simulink model "Diesel_NGCHP_v2"  (Simulink 8.1)
settings: Solver=ode4  StartTime=0.0  StopTime=inf  FixedStep=Ts  MaxStep=1e-3  RelTol=1e-3
model workspace (MAT data in the model file):
  op_snapshot1 : opcond.OperatingPoint (value not decoded)
PostLoadFcn:
  | Diesel_NGCHP_init;
InitFcn:
  | Diesel_NGCHP_init;
values from neighbouring files (symbols this model uses):
  Ts = 100E-6    (= 0.0001)    [Diesel_NGCHP_init.m]
undefined symbols (not defined in the file or in its folder): cable_spec, Diesel_Genset_lib, DiscIntNeverNeededParam, fdesignblkfcn, gcbh, Left, NG_CHP, NG_CHP_lib, ph, type, V
libraries: simulink x16, rtio_opalrt_common x15, powerlib x11, NG_Genset_lib x6, cables_lib x6, rtlab x5, simulink_extras x5, breaker_lib x4, rteventslib x4, powerlib_extras x3, discretizing x2, ssn_lib x2
(part 1 of 3)
settings Model: ARTEMISmethode_block_infos=$$__separator__$$Diesel_NGCHP_v2/ARTEMIS Guide$$__separator__$$  Creator=RE25624  LastModifiedBy=re25624  BufferReuse=off
settings SolverCC: ZeroCrossAlgorithm=Adaptive
settings DataIOCC: ExternalInput=getinputstruct(op_snapshot1)  InitialState=getstatestruct(op_snapshot1)  LimitDataPoints=off  MaxDataPoints=90060  SignalLoggingSaveFormat=Dataset  SaveOutput=off  SignalLogging=off  DSMLogging=off  SaveTime=off  OutputSaveName=result
settings OptimizationCC: BlockReduction=off  OptimizeBlockIOStorage=off  BufferReuse=off  ExpressionFolding=off  LocalBlockOutputs=off
settings DebuggingCC: MaxConsecutiveZCsMsg=warning  IgnoredZcDiagnostic=none  SolverPrmCheckMsg=none  MultiTaskRateTransMsg=warning  FcnCallInpInsideContextMsg=EnableAllAsWarning  FrameProcessingCompatibilityMsg=error  ModelReferenceExtraNoncontSigs=warning  StrictBusMsg=None
settings ModelReferenceCC: UpdateModelReferenceTargets=IfOutOfDate
settings SFSimCC: SFSimEcho=off
settings GRTTargetCC: CodeReplacementLibrary=C89/C90 (ANSI)

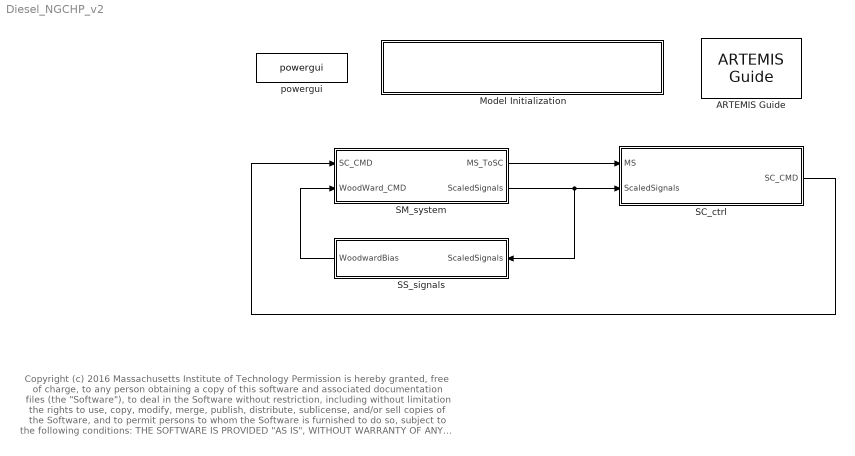
== system Diesel_NGCHP_v2 ==
  note: Copyright (c) 2016 Massachusetts Institute of Technology
      | Permission is hereby granted, free of charge, to any person obtaining a copy of this software and associated documentation files (the "Software"), to deal
      | in the Software without restriction, including without limitation the rights to use, copy, modify, merge, publish, distribute, sublicense, and/or sell copies of the
      | Software, and to permit persons to whom the Software is furnished to do so, subject to the following conditions:
      |
      | THE SOFTWARE IS PROVIDED "AS IS", WITHOUT WARRANTY OF ANY KIND, EXPRESS OR IMPLIED, INCLUDING BUT NOT LIMITED TO THE
      | WARRANTIES OF MERCHANTABILITY, FITNESS FOR A PARTICULAR PURPOSE AND NONINFRINGEMENT. IN NO EVENT SHALL THE AUTHORS
      | OR COPYRIGHT HOLDERS BE LIABLE FOR ANY CLAIM, DAMAGES OR OTHER LIABILITY, WHETHER IN AN ACTION OF CONTRACT, TORT OR
      | OTHERWISE, ARISING FROM, OUT OF OR IN CONNECTION WITH THE SOFTWARE OR THE USE OR OTHER DEALINGS IN THE SOFTWARE.
  ARTEMIS Guide : artemis/ARTEMIS/ARTEMIS Guide  Tag=FTSSmethode_opal_4hx0r99  Description=5.0_z1  lock=on  Ts=Ts  opt=art5  dyna=off  nb_perm=4  RT_fullcomp=off  ssn=on  ssn_itvc=off  ssn_ivic=off  ssn_ext=off  ssn_solver=Art5 with Backward Euler nodal interface  ssn_impulse=off  ssn_quasimpulse=off  ssn_impulse_loop=2  paraExtinctionThy=off  Thy_Impulse=on  dtc=Off  dtc_opt=normal  ao=on  simtype=off  ct_mac=off  lin_mov=off  lsp=[0.001 2]  spike_skip=Disabled  dtc_extra=1  dtc_sws=normal  dtc_pied=0.5  SPSRulesBlock=SPSRules  tre=on  ctmm=off  LF=off  dpl_type=ARTEMiS DPL  rlc_type=off  custom_type=off  para=on  ssn_ImpulseLoopBlockedStateUpdate=2  ssn_mov_iter_number=5  ssn_switch_iter_number=5
  Model Initialization : Subsystem  AncestorBlock=artemis/Tools /Misc/Model Initialization  mask(Model Functions){InitFcnX=Diesel_NGCHP_init;, prel=off, posl=on, inif=on, strf=off}
      mask prompts: InitFcnX "Initialisation"; prel "Preload Function"; posl "PostLoad Function"; inif "InitFcn"; strf "StartFcn"
      mask init:
      | currentBlock = gcb;
      | root = bdroot(currentBlock);
      | 
      | 
      | if ~strcmp(get_param(root,'BlockDiagramType'),'library')
      |     if prel==1
      |         set_param(root, 'PreLoadFcn', InitFcnX);
      |     else
      |         set_param(root, 'PreLoadFcn', '');
      |     end
      |     if inif==1
      |         set_param(root, 'InitFcn', InitFcnX);
      |     else
      |         set_param(root, 'InitFcn', '');
      |     end
      |     if strf==1
      |         set_param(root, 'StartFcn', InitFcnX);
      |     else
      |         set_param(root, 'StartFcn', '');
      |     end
      |     if posl==1
      |         set_param(root, 'PostLoadFcn', InitFcnX);
      |     else
      |         set_param(root, 'PostLoadFcn', '');
      |     end
      | end
      | 
      | pos = get_param(currentBlock, 'Position');
      | width = pos(3) - pos(1); height = pos(4) - pos(2);
      | txt = [ upper(root) '\n' '- InitFcn. . . . . '  get_param(root, 'InitFcn') ];
      settings: CopyFcn=set_param(gcb,'LinkStatus','inactive')
      mask Display: text(5, height*0.5, txt, 'horizontalAlignment', 'left', 'verticalAlignment', 'middle') ;
  SC_ctrl : Subsystem
  SM_system : Subsystem
  SS_signals : Subsystem
  powergui : powerlib/powergui  Priority=2  SimulationMode=Discrete  SolverType=Tustin  SampleTime=Ts  frequency=60  SPID=off  DisableSnubberDevices=off  DisableRonSwitches=off  DisableVfSwitches=off  SwTol=0  Interpol=off  DisplayEquations=off  frequencyindice=0  Pbase=100e6  ErrMax=1e-4  Iterations=50  UnitsV=kV  UnitsW=MW  FunctionMessages=off  echomessages=off  HookPort=off  EnableUseOfTLC=off  x0status=blocks  RestoreLinks=warning  ResistiveCurrentMeasurement=off  Frange=logspace(0,3,50)  Ylog=off  Xlog=off  ShowGrid=off  save=off  variable=ZData  structure=0  ZoomFFT=on  StartTime=0.0  cycles=2  DisplayStyle=off  fundamental=60  FreqAxis=off  MaxFrequency=1000  frequencyindicesteady=1  RmsSteady=1  display=off  Ts=0  methode=off
  wires:
  SM_system/1(MS_ToSC) -> SC_ctrl/1(MS)
  SC_ctrl/1(SC_CMD) -> SM_system/1(SC_CMD)
  SM_system/2(ScaledSignals) -> SS_signals/1(ScaledSignals), SC_ctrl/2(ScaledSignals)
  SS_signals/1(WoodwardBias) -> SM_system/2(WoodWard_CMD)

== system Diesel_NGCHP_v2/Model Initialization ==

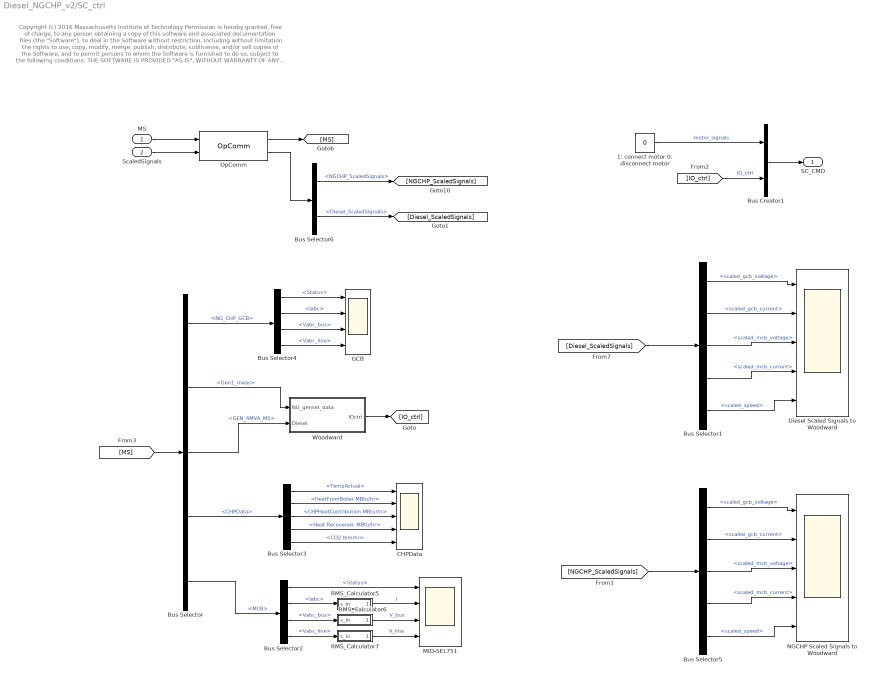
== system Diesel_NGCHP_v2/SC_ctrl ==
  note: Copyright (c) 2016 Massachusetts Institute of Technology
      | Permission is hereby granted, free of charge, to any person obtaining a copy of this software and associated documentation files (the "Software"), to deal
      | in the Software without restriction, including without limitation the rights to use, copy, modify, merge, publish, distribute, sublicense, and/or sell copies of the
      | Software, and to permit persons to whom the Software is furnished to do so, subject to the following conditions:
      |
      | THE SOFTWARE IS PROVIDED "AS IS", WITHOUT WARRANTY OF ANY KIND, EXPRESS OR IMPLIED, INCLUDING BUT NOT LIMITED TO THE
      | WARRANTIES OF MERCHANTABILITY, FITNESS FOR A PARTICULAR PURPOSE AND NONINFRINGEMENT. IN NO EVENT SHALL THE AUTHORS
      | OR COPYRIGHT HOLDERS BE LIABLE FOR ANY CLAIM, DAMAGES OR OTHER LIABILITY, WHETHER IN AN ACTION OF CONTRACT, TORT OR
      | OTHERWISE, ARISING FROM, OUT OF OR IN CONNECTION WITH THE SOFTWARE OR THE USE OR OTHER DEALINGS IN THE SOFTWARE
  MS : Inport
  ScaledSignals : Inport  Port=2
  1: connect motor 0: disconnect motor : Constant  Value=0
  Bus Creator1 : BusCreator  Inputs=2
  Bus Selector : BusSelector  OutputSignals=NG_CHP_MS.NG_CHP_GCB,NG_CHP_MS.Gen1_meas,GEN_4MVA_MS,NG_CHP_MS.CHPData,MCB
  Bus Selector1 : BusSelector  OutputSignals=scaled_gcb_voltage,scaled_gcb_current,scaled_mcb_voltage,scaled_mcb_current,scaled_speed
  Bus Selector2 : BusSelector  OutputSignals=Status,Iabc,Vabc_bus,Vabc_line
  Bus Selector3 : BusSelector  OutputSignals=TempActual,HeatFromBoiler MBtu/hr,CHPHeatContribution MBtu/hr,Thermal data.Heat Recovered; MBtu/hr,Thermal data.CO2 lbm/hr
  Bus Selector4 : BusSelector  OutputSignals=Status,Iabc,Vabc_bus,Vabc_line
  Bus Selector5 : BusSelector  OutputSignals=scaled_gcb_voltage,scaled_gcb_current,scaled_mcb_voltage,scaled_mcb_current,scaled_speed
  Bus Selector6 : BusSelector  OutputSignals=NGCHP_ScaledSignals,Diesel_ScaledSignals
  CHPData : Scope  NumInputPorts=5
      settings: ShowLegends=on  TimeRange=10  YMin=19.11~0~-1~1.37518~932.98  YMax=19.2~5.5~1~1.37533~933.08  SaveName=ScopeData5
  Diesel Scaled Signals to Woodward : Scope  NumInputPorts=5
      settings: YMin=-17.5~-0.000175~-17.5~-45~-5  YMax=17.5~0.000175~17.5~45~10  SaveName=ScopeData7
  GCB : Scope  NumInputPorts=4
      settings: ShowLegends=on  TimeRange=0.02  YMin=-1~-0.00015~-0.0025~-12500  YMax=1~0.00015~0.0025~12500
  MID-SEL751 : Scope  NumInputPorts=4
      settings: ShowLegends=on  TimeRange=1  YMin=0.95~-225~-12000~-12000  YMax=1.05~225~12000~12000  SaveName=ScopeData2
  NGCHP Scaled Signals to Woodward : Scope  NumInputPorts=5
      settings: YMin=-17.5~-0.000175~-17.5~-45~-5  YMax=17.5~0.000175~17.5~45~10  SaveName=ScopeData8
  OpComm : rtlab/OpComm  nbport=2  groupe_acq=1  subsys_rate=0  st=0  Synchronization=on  Interpolation=on  Threshold=1.0  Missed_Data=off  Sim_Time=off  Samples=off  dynSigOut=off  from_console=0  warning_done=off  writeOpCommFile=off  Offset=off
  RMS_Calculator5 : Subsystem
  RMS_Calculator6 : Subsystem
  RMS_Calculator7 : Subsystem
  Woodward : Subsystem
  SC_CMD : Outport
  wires:
  OpComm/1 -> [MS]
  MS/1 -> OpComm/1
  Woodward/1(IOctrl) -> [IO_ctrl]
  Bus Selector4/1 -> GCB/1  "<Status>"
  Bus Selector4/2 -> GCB/2  "<Iabc>"
  Bus Selector4/3 -> GCB/3  "<Vabc_bus>"
  Bus Selector4/4 -> GCB/4  "<Vabc_line>"
  Bus Selector/1 -> Bus Selector4/1  "<NG_CHP_GCB>"
  Bus Selector/2 -> Woodward/1(NG_genset_data)  "<Gen1_meas>"
  [MS] -> Bus Selector/1
  Bus Selector/4 -> Bus Selector3/1  "<CHPData>"
  Bus Selector3/1 -> CHPData/1  "<TempActual>"
  Bus Selector3/5 -> CHPData/5  "<CO2 lbm/hr>"
  Bus Selector3/2 -> CHPData/2  "<HeatFromBoiler MBtu/hr>"
  Bus Selector3/3 -> CHPData/3  "<CHPHeatContribution MBtu/hr>"
  Bus Selector3/4 -> CHPData/4  "<Heat Recovered; MBtu/hr>"
  Bus Creator1/1 -> SC_CMD/1
  1: connect motor 0: disconnect motor/1 -> Bus Creator1/1  "motor_signals"
  Bus Selector2/1 -> MID-SEL751/1  "<Status>"
  Bus Selector2/2 -> RMS_Calculator5/1(s_in)  "<Iabc>"
  Bus Selector2/3 -> RMS_Calculator6/1(s_in)  "<Vabc_bus>"
  Bus Selector2/4 -> RMS_Calculator7/1(s_in)  "<Vabc_line>"
  RMS_Calculator5/1(s_out) -> MID-SEL751/2  "I"
  RMS_Calculator6/1(s_out) -> MID-SEL751/3  "V_bus"
  RMS_Calculator7/1(s_out) -> MID-SEL751/4  "V_line"
  Bus Selector/5 -> Bus Selector2/1  "<MCB>"
  Bus Selector/3 -> Woodward/2(Diesel)  "<GEN_4MVA_MS>"
  [IO_ctrl] -> Bus Creator1/2  "IO_ctrl"
  Bus Selector1/1 -> Diesel Scaled Signals to Woodward/1  "<scaled_gcb_voltage>"
  Bus Selector1/2 -> Diesel Scaled Signals to Woodward/2  "<scaled_gcb_current>"
  Bus Selector1/3 -> Diesel Scaled Signals to Woodward/3  "<scaled_mcb_voltage>"
  Bus Selector1/4 -> Diesel Scaled Signals to Woodward/4  "<scaled_mcb_current>"
  Bus Selector1/5 -> Diesel Scaled Signals to Woodward/5  "<scaled_speed>"
  [Diesel_ScaledSignals] -> Bus Selector1/1
  Bus Selector5/1 -> NGCHP Scaled Signals to Woodward/1  "<scaled_gcb_voltage>"
  Bus Selector5/2 -> NGCHP Scaled Signals to Woodward/2  "<scaled_gcb_current>"
  Bus Selector5/3 -> NGCHP Scaled Signals to Woodward/3  "<scaled_mcb_voltage>"
  Bus Selector5/4 -> NGCHP Scaled Signals to Woodward/4  "<scaled_mcb_current>"
  Bus Selector5/5 -> NGCHP Scaled Signals to Woodward/5  "<scaled_speed>"
  [NGCHP_ScaledSignals] -> Bus Selector5/1
  OpComm/2 -> Bus Selector6/1
  Bus Selector6/1 -> [NGCHP_ScaledSignals]  "<NGCHP_ScaledSignals>"
  Bus Selector6/2 -> [Diesel_ScaledSignals]  "<Diesel_ScaledSignals>"
  ScaledSignals/1 -> OpComm/2

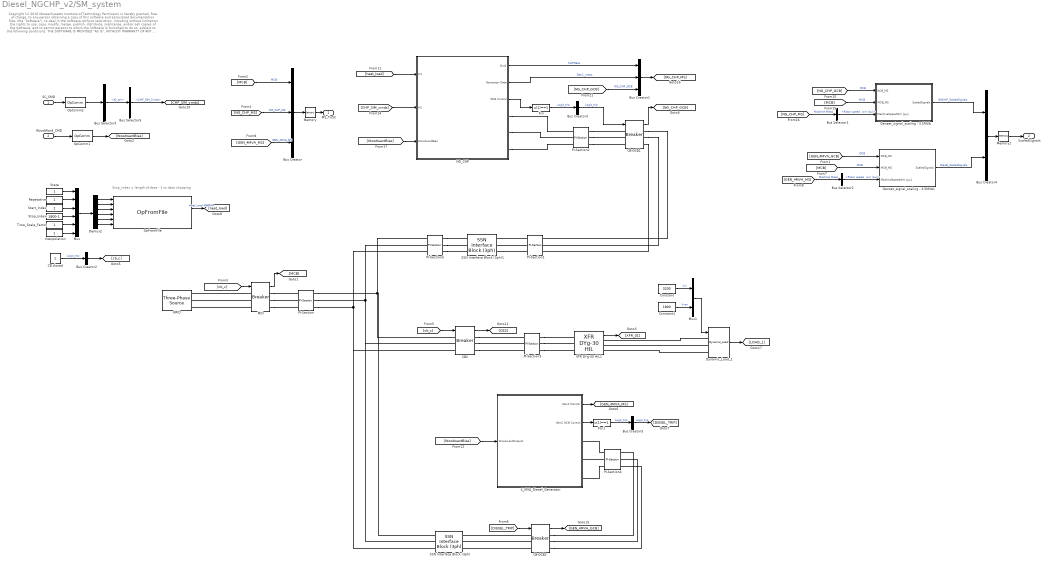
== system Diesel_NGCHP_v2/SM_system ==
  note: Copyright (c) 2016 Massachusetts Institute of Technology
      | Permission is hereby granted, free of charge, to any person obtaining a copy of this software and associated documentation files (the "Software"), to deal
      | in the Software without restriction, including without limitation the rights to use, copy, modify, merge, publish, distribute, sublicense, and/or sell copies of the
      | Software, and to permit persons to whom the Software is furnished to do so, subject to the following conditions:
      |
      | THE SOFTWARE IS PROVIDED "AS IS", WITHOUT WARRANTY OF ANY KIND, EXPRESS OR IMPLIED, INCLUDING BUT NOT LIMITED TO THE
      | WARRANTIES OF MERCHANTABILITY, FITNESS FOR A PARTICULAR PURPOSE AND NONINFRINGEMENT. IN NO EVENT SHALL THE AUTHORS
      | OR COPYRIGHT HOLDERS BE LIABLE FOR ANY CLAIM, DAMAGES OR OTHER LIABILITY, WHETHER IN AN ACTION OF CONTRACT, TORT OR
      | OTHERWISE, ARISING FROM, OUT OF OR IN CONNECTION WITH THE SOFTWARE OR THE USE OR OTHER DEALINGS IN THE SOFTWARE
  note: Stop_index = length of data - 1 to data chopping
  SC_CMD : Inport
  WoodWard_CMD : Inport  Port=2
  4_MVA_Diesel_Generator : Subsystem  AncestorBlock=Diesel_Genset_lib/4_MVA_Diesel_Generator
  Bus Creator : BusCreator  Inputs=3
  Bus Creator1 : BusCreator  Inputs=3
  Bus Creator2 : BusCreator  Inputs=1
  Bus Creator3 : BusCreator  Inputs=1
  Bus Creator4 : BusCreator  Inputs=2
  Bus Creator5 : BusCreator  Inputs=1
  Bus Selector1 : BusSelector  OutputSignals="Gen1_meas.w.w.Rotor speed  wm (pu)"
  Bus Selector2 : BusSelector  OutputSignals="w.w.Rotor speed  wm (pu)"
  Bus Selector3 : BusSelector  OutputSignals=IO_ctrl
  Bus Selector5 : BusSelector  OutputSignals=16 DOUT GR3.CHP_SIM_Cmds
  CB closed : Constant
  CB-GCB1 : breaker_lib/Breaker  Ts=Ts  mech_delay=cb_mech_delay
  CB-GCB2 : breaker_lib/Breaker  Ts=Ts  mech_delay=cb_mech_delay
  CB2 : breaker_lib/Breaker  Ts=Ts  mech_delay=cb_mech_delay
  Constant : Constant  Value=3200
  Constant1 : Constant  Value=1800
  Demux2 : Demux  Outputs=6
  Dynamic_Load_1 : Load_lib/Dynamic_Load  V=4160  Ts=Ts
  Fcn : Fcn  Expr=u(1)==1
  Fcn1 : Fcn  Expr=u(1)==1
  GRID : powerlib/Electrical Sources/Three-Phase Source  Voltage=13800  PhaseAngle=0  Frequency=60  InternalConnection=Yg  SpecifyImpedance=on  Resistance=0.8929  Inductance=16.58e-3  ShortCircuitLevel=375e6  BaseVoltage=13800  XRratio=4.6  BusType=swing  Pref=0  Qref=0  Qmin=-inf  Qmax=inf
  Genset_signal_scaling - 3.5MVA : Subsystem  mask(Genset Signal Scaling for Opal-RT/Woodward){Vpk_mcb=11268, watt_mcb=3150000, Vpk_gcb=11268, watt_gcb=3150000, rated_rpm=1800, wm_noise_bias=0.02}
      mask prompts: Vpk_mcb "MCB Nominal Voltage [Vpk]"; watt_mcb "MCB Watts [W]"; Vpk_gcb "GCB Nominal Voltage [ Vpk]"; watt_gcb "GCB Watts [W]"; rated_rpm "Machine Rated Speed [RPM]"; wm_noise_bias "Speed Noise Bias [0-1]"
      mask help:
      | Scaling for voltages:
      | For 120 => 12Vout / 170Vpk
      | For 480 => 12Vout / 391Vpk
      | For 13.8kv => 12Vout / 11268Vpk
      |
      | Scaling for currents - used in the 1 MVA genset:
      | 15Vout / ( 900000W / 391Vpk)
      |
      | Scaling for currents - used in the 3.5 MVA NG/CHP:
      | 15Vout / ( 3150000W / 11268Vpk)
      | - Current scale factors chosen to match easYgen settings for 3.5 MVA gas engine CT ratio of 1500/x made on 20160508
  Genset_signal_scaling - 3.5MVA1 : Subsystem  mask(Genset Signal Scaling for Opal-RT/Woodward){Vpk_mcb=11268, watt_mcb=3150000, Vpk_gcb=11268, watt_gcb=3150000, rated_rpm=1800, wm_noise_bias=0.02}
      mask prompts: Vpk_mcb "MCB Nominal Voltage [Vpk]"; watt_mcb "MCB Watts [W]"; Vpk_gcb "GCB Nominal Voltage [ Vpk]"; watt_gcb "GCB Watts [W]"; rated_rpm "Machine Rated Speed [RPM]"; wm_noise_bias "Speed Noise Bias [0-1]"
      mask help:
      | Scaling for voltages:
      | For 120 => 12Vout / 170Vpk
      | For 480 => 12Vout / 391Vpk
      | For 13.8kv => 12Vout / 11268Vpk
      |
      | Scaling for currents - used in the 1 MVA genset:
      | 15Vout / ( 900000W / 391Vpk)
      |
      | Scaling for currents - used in the 3.5 MVA NG/CHP:
      | 15Vout / ( 3150000W / 11268Vpk)
      | - Current scale factors chosen to match easYgen settings for 3.5 MVA gas engine CT ratio of 1500/x made on 20160508
  "Interpolation " : Constant
  MID : breaker_lib/Breaker  Ts=Ts  mech_delay=cb_mech_delay
  Memory : Memory
  Memory1 : Memory
  Mux : Mux  Inputs=6
  Mux1 : Mux  Inputs=2
  NG_CHP : Subsystem  AncestorBlock=NG_CHP_lib/NG_CHP
  OpComm1 : rtlab/OpComm  nbport=1  groupe_acq=1  subsys_rate=0  st=0  Synchronization=on  Interpolation=on  Threshold=1.0  Missed_Data=off  Sim_Time=off  Samples=off  dynSigOut=off  from_console=0  warning_done=off  writeOpCommFile=off  Offset=off
  OpComm2 : rtlab/OpComm  nbport=1  groupe_acq=1  subsys_rate=0  st=0  Synchronization=on  Interpolation=on  Threshold=1.0  Missed_Data=off  Sim_Time=off  Samples=off  dynSigOut=off  from_console=1  warning_done=off  writeOpCommFile=off  Offset=off
  OpFromFile : rtlab/DataLogging/OpFromFile  filename_mode=Static (same filename all the time)  reload_mode=Next time model is paused (Real-Time)  init_file_id=0  filename=HeatLoad.mat  rtpath='./'  nrtpath='.\'  sample_time=Ts
  PI-Section : cables_lib/PI-Section  cable_spec=[cable_spec(13, :)]  line_length=5500  parallel_sets=1
  PI-Section1 : cables_lib/PI-Section  cable_spec=[cable_spec(11, :)]  line_length=10  parallel_sets=1
  PI-Section2 : cables_lib/PI-Section  cable_spec=[cable_spec(11, :)]  line_length=2000  parallel_sets=1
  PI-Section3 : cables_lib/PI-Section  cable_spec=[cable_spec(13, :)]  line_length=1500  parallel_sets=1
  PI-Section4 : cables_lib/PI-Section  cable_spec=[cable_spec(11, :)]  line_length=2000  parallel_sets=1
  PI-Section5 : cables_lib/PI-Section  cable_spec=[cable_spec(11, :)]  line_length=10  parallel_sets=1
  "Repetative " : Constant
  SSN Interface Block (3ph) : ssn_lib/SSN Interface Block (3ph)  nb_phase=3  nb_port=2  p1_type=V-type(Left)  p2_type=V-type (Right)  p3_type=V-type(Left)  p4_type=V-type(Left)  p5_type=V-type(Left)  p6_type=V-type(Left)  p7_type=V-type(Left)  p8_type=V-type(Left)  p9_type=V-type(Left)  p10_type=V-type(Left)  p11_type=V-type(Left)  p12_type=V-type(Left)  p13_type=V-type(Left)  p14_type=V-type(Left)  p15_type=V-type(Left)  p16_type=V-type(Left)  I_port_shunt_resistance=1e9
  SSN Interface Block (3ph)1 : ssn_lib/SSN Interface Block (3ph)  nb_phase=3  nb_port=2  p1_type=V-type(Left)  p2_type=V-type (Right)  p3_type=V-type(Left)  p4_type=V-type(Left)  p5_type=V-type(Left)  p6_type=V-type(Left)  p7_type=V-type(Left)  p8_type=V-type(Left)  p9_type=V-type(Left)  p10_type=V-type(Left)  p11_type=V-type(Left)  p12_type=V-type(Left)  p13_type=V-type(Left)  p14_type=V-type(Left)  p15_type=V-type(Left)  p16_type=V-type(Left)  I_port_shunt_resistance=1e9
  "Start_Index " : Constant
  "State " : Constant
  "Stop_Index " : Constant  Value=1800-1
  "Time_Scale_Factor " : Constant
  XFR DYg-30 HIL1 : transformer_lib/XFR DYg-30 HIL  Rating=3750  Vp=13800  Vs=4160  Z=4.75  XR=11.4
  MS_ToSC : Outport
  ScaledSignals : Outport  Port=2
  wires:
  MID/1 -> [MCB]
  Bus Creator/1 -> Memory/1
  CB-GCB1/1 -> [NG_CHP_GCB]
  SC_CMD/1 -> OpComm2/1
  [NG_CHP_GCB] -> Bus Creator1/3  "NG_CHP_GCB"
  NG_CHP/2(Generator Data) -> Bus Creator1/2  "Gen1_meas"
  XFR DYg-30 HIL1/1 -> [XFR_01]
  "Stop_Index "/1 -> Mux/4
  "Interpolation "/1 -> Mux/6
  "Start_Index "/1 -> Mux/3
  "Time_Scale_Factor "/1 -> Mux/5
  "Repetative "/1 -> Mux/2
  "State "/1 -> Mux/1
  NG_CHP/1(Out1) -> Bus Creator1/1  "CHPData"
  NG_CHP/3(GCB Control) -> Fcn/1
  Bus Selector5/1 -> [CHP_SIM_cmds]  "<CHP_SIM_Cmds>"
  OpFromFile/2 -> [heat_load]  "Heat Load MBtu/hr"
  [heat_load] -> NG_CHP/1(In1)
  [CHP_SIM_cmds] -> NG_CHP/2(In2)
  Demux2/2 -> OpFromFile/2
  Demux2/5 -> OpFromFile/5
  Demux2/4 -> OpFromFile/4
  Demux2/1 -> OpFromFile/1
  Demux2/6 -> OpFromFile/6
  Demux2/3 -> OpFromFile/3
  Dynamic_Load_1/1 -> [LOAD_1]
  Bus Creator2/1 -> [cb_c]
  CB closed/1 -> Bus Creator2/1  "Logic_trip"
  CB2/1 -> [CB2]
  [MCB] -> Bus Creator/1  "MCB"
  [GEN_4MVA_MS] -> Bus Creator/3  "GEN_4MVA_MS"
  Bus Creator1/1 -> [NG_CHP_MS]
  [NG_CHP_MS] -> Bus Creator/2  "NG_CHP_MS"
  Mux/1 -> Demux2/1
  Mux1/1 -> Dynamic_Load_1/1
  Fcn/1 -> Bus Creator3/1  "Logic_trip"
  Bus Creator3/1 -> CB-GCB1/1  "Logic_trip"
  [cb_c] -> MID/1
  OpComm2/1 -> Bus Selector3/1
  Bus Selector3/1 -> Bus Selector5/1  "<IO_ctrl>"
  Memory/1 -> MS_ToSC/1
  Constant1/1 -> Mux1/2  "kvar"
  Constant/1 -> Mux1/1  "kw"
  [cb_c] -> CB2/1
  CB-GCB2/1 -> [GEN_4MVA_GCB]
  [DIESEL_TRIP] -> CB-GCB2/1
  4_MVA_Diesel_Generator/1(Gen2 Monitor) -> [GEN_4MVA_MS]
  4_MVA_Diesel_Generator/2(Gen2 GCB Control) -> Fcn1/1
  Fcn1/1 -> Bus Creator5/1  "Logic_trip"
  Bus Creator5/1 -> [DIESEL_TRIP]  "Logic_trip"
  [GEN_4MVA_MS] -> Bus Selector2/1  "Machine Meas"
  [GEN_4MVA_GCB] -> Genset_signal_scaling - 3.5MVA1/1(GCB_MS)  "GCB"
  [MCB] -> Genset_signal_scaling - 3.5MVA1/2(MCB_MS)  "MCB"
  Bus Selector2/1 -> Genset_signal_scaling - 3.5MVA1/3(MachineSpeedWm [pu])  "<Rotor speed  wm (pu)>"
  [NG_CHP_MS] -> Bus Selector1/1  "Machine Meas"
  [NG_CHP_GCB] -> Genset_signal_scaling - 3.5MVA/1(GCB_MS)  "GCB"
  [MCB] -> Genset_signal_scaling - 3.5MVA/2(MCB_MS)  "MCB"
  Bus Selector1/1 -> Genset_signal_scaling - 3.5MVA/3(MachineSpeedWm [pu])  "<Rotor speed  wm (pu)>"
  Bus Creator4/1 -> Memory1/1
  Memory1/1 -> ScaledSignals/1
  Genset_signal_scaling - 3.5MVA/1(ScaledSignals) -> Bus Creator4/1  "NGCHP_ScaledSignals"
  Genset_signal_scaling - 3.5MVA1/1(ScaledSignals) -> Bus Creator4/2  "Diesel_ScaledSignals"
  WoodWard_CMD/1 -> OpComm1/1
  OpComm1/1 -> [WoodwardBias]
  [WoodwardBias] -> NG_CHP/3(WoodwardBias)
  [WoodwardBias] -> 4_MVA_Diesel_Generator/1(WoodwardOutputs)
  connections:
  Dynamic_Load_1/LConn1 -- XFR DYg-30 HIL1/RConn1
  Dynamic_Load_1/LConn2 -- XFR DYg-30 HIL1/RConn2
  Dynamic_Load_1/LConn3 -- XFR DYg-30 HIL1/RConn3
  CB2/RConn2 -- PI-Section3/LConn2
  CB2/RConn1 -- PI-Section3/LConn1
  CB2/RConn3 -- PI-Section3/LConn3
  PI-Section5/LConn3 -- SSN Interface Block (3ph)/LConn3 -- CB2/LConn3 -- PI-Section/RConn3
  PI-Section5/LConn2 -- SSN Interface Block (3ph)/LConn2 -- CB2/LConn2 -- PI-Section/RConn2
  PI-Section5/LConn1 -- SSN Interface Block (3ph)/LConn1 -- CB2/LConn1 -- PI-Section/RConn1
  PI-Section3/RConn2 -- XFR DYg-30 HIL1/LConn2
  PI-Section3/RConn3 -- XFR DYg-30 HIL1/LConn3
  PI-Section3/RConn1 -- XFR DYg-30 HIL1/LConn1
  PI-Section2/RConn3 -- CB-GCB1/LConn3
  PI-Section2/RConn2 -- CB-GCB1/LConn2
  PI-Section2/RConn1 -- CB-GCB1/LConn1
  NG_CHP/RConn2 -- PI-Section2/LConn2
  NG_CHP/RConn3 -- PI-Section2/LConn3
  NG_CHP/RConn1 -- PI-Section2/LConn1
  PI-Section1/LConn1 -- SSN Interface Block (3ph)1/RConn1
  PI-Section1/LConn2 -- SSN Interface Block (3ph)1/RConn2
  PI-Section1/LConn3 -- SSN Interface Block (3ph)1/RConn3
  PI-Section5/RConn2 -- SSN Interface Block (3ph)1/LConn2
  PI-Section5/RConn1 -- SSN Interface Block (3ph)1/LConn1
  PI-Section5/RConn3 -- SSN Interface Block (3ph)1/LConn3
  CB-GCB1/RConn3 -- PI-Section1/RConn3
  CB-GCB1/RConn1 -- PI-Section1/RConn1
  CB-GCB1/RConn2 -- PI-Section1/RConn2
  MID/RConn3 -- PI-Section/LConn3
  MID/RConn2 -- PI-Section/LConn2
  MID/RConn1 -- PI-Section/LConn1
  MID/LConn3 -- GRID/RConn3
  MID/LConn1 -- GRID/RConn1
  MID/LConn2 -- GRID/RConn2
  CB-GCB2/RConn3 -- PI-Section4/RConn3
  CB-GCB2/RConn2 -- PI-Section4/RConn2
  CB-GCB2/RConn1 -- PI-Section4/RConn1
  PI-Section4/LConn3 -- 4_MVA_Diesel_Generator/RConn3
  PI-Section4/LConn2 -- 4_MVA_Diesel_Generator/RConn2
  PI-Section4/LConn1 -- 4_MVA_Diesel_Generator/RConn1
  CB-GCB2/LConn3 -- SSN Interface Block (3ph)/RConn3
  CB-GCB2/LConn1 -- SSN Interface Block (3ph)/RConn1
  CB-GCB2/LConn2 -- SSN Interface Block (3ph)/RConn2

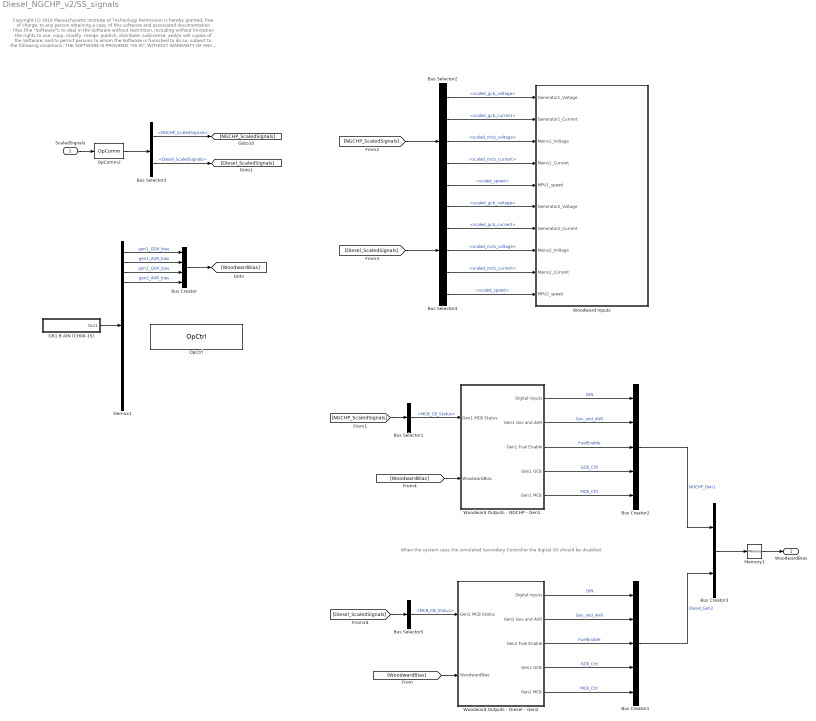
== system Diesel_NGCHP_v2/SS_signals ==
  note: Copyright (c) 2016 Massachusetts Institute of Technology
      | Permission is hereby granted, free of charge, to any person obtaining a copy of this software and associated documentation files (the "Software"), to deal
      | in the Software without restriction, including without limitation the rights to use, copy, modify, merge, publish, distribute, sublicense, and/or sell copies of the
      | Software, and to permit persons to whom the Software is furnished to do so, subject to the following conditions:
      |
      | THE SOFTWARE IS PROVIDED "AS IS", WITHOUT WARRANTY OF ANY KIND, EXPRESS OR IMPLIED, INCLUDING BUT NOT LIMITED TO THE
      | WARRANTIES OF MERCHANTABILITY, FITNESS FOR A PARTICULAR PURPOSE AND NONINFRINGEMENT. IN NO EVENT SHALL THE AUTHORS
      | OR COPYRIGHT HOLDERS BE LIABLE FOR ANY CLAIM, DAMAGES OR OTHER LIABILITY, WHETHER IN AN ACTION OF CONTRACT, TORT OR
      | OTHERWISE, ARISING FROM, OUT OF OR IN CONNECTION WITH THE SOFTWARE OR THE USE OR OTHER DEALINGS IN THE SOFTWARE
  note: When the system uses the simulated
      | Secondary Controller the digital I/O
      | should be disabled.
  ScaledSignals : Inport
  Bus Creator : BusCreator
  Bus Creator1 : BusCreator  Inputs=5
  Bus Creator2 : BusCreator  Inputs=5
  Bus Creator3 : BusCreator  Inputs=2
  Bus Selector1 : BusSelector  OutputSignals=MCB_CB_Status
  Bus Selector2 : BusSelector  OutputSignals=scaled_gcb_voltage,scaled_gcb_current,scaled_mcb_voltage,scaled_mcb_current,scaled_speed
  Bus Selector3 : BusSelector  OutputSignals=NGCHP_ScaledSignals,Diesel_ScaledSignals
  Bus Selector4 : BusSelector  OutputSignals=scaled_gcb_voltage,scaled_gcb_current,scaled_mcb_voltage,scaled_mcb_current,scaled_speed
  Bus Selector5 : BusSelector  OutputSignals=MCB_CB_Status
  Demux1 : Demux  Outputs=16
  GR1 B AIN (CH00-15) : Subsystem
  Memory1 : Memory
  OpComm2 : rtlab/OpComm  nbport=1  groupe_acq=1  subsys_rate=0  st=0  Synchronization=on  Interpolation=on  Threshold=1.0  Missed_Data=off  Sim_Time=off  Samples=off  dynSigOut=off  from_console=0  warning_done=off  writeOpCommFile=off  Offset=off
  OpCtrl : rtio_opalrt_common/OpCtrl  CtrlName='OpCtrl'  boardid=0  BitstreamFilename=VC707_2-EX-0001-2_2_6_61-32AIO16DIO16DIOSel-01-01.bin  numconfig=-1  mode=Master  externalClock=off  decimRtsi=0  calibIO=off  SampleTime=0  loadinport=-1  BoardType=VC707  SecondaryPresent=off  sync_type=Audio
  Woodward Inputs : Subsystem
  Woodward Outputs - Diesel - Gen2 : Subsystem
  Woodward Outputs - NGCHP - Gen1 : Subsystem
  WoodwardBias : Outport
  wires:
  ScaledSignals/1 -> OpComm2/1
  OpComm2/1 -> Bus Selector3/1
  Bus Selector3/1 -> [NGCHP_ScaledSignals]  "<NGCHP_ScaledSignals>"
  Bus Selector3/2 -> [Diesel_ScaledSignals]  "<Diesel_ScaledSignals>"
  [NGCHP_ScaledSignals] -> Bus Selector2/1
  Bus Selector2/5 -> Woodward Inputs/5(MPU1_speed)  "<scaled_speed>"
  Bus Selector2/4 -> Woodward Inputs/4(Mains1_Current)  "<scaled_mcb_current>"
  Bus Selector2/3 -> Woodward Inputs/3(Mains1_Voltage)  "<scaled_mcb_voltage>"
  Bus Selector2/2 -> Woodward Inputs/2(Generator1_Current)  "<scaled_gcb_current>"
  Bus Selector2/1 -> Woodward Inputs/1(Generator1_Voltage)  "<scaled_gcb_voltage>"
  [Diesel_ScaledSignals] -> Bus Selector4/1
  Bus Selector4/1 -> Woodward Inputs/6(Generator2_Voltage)  "<scaled_gcb_voltage>"
  Bus Selector4/2 -> Woodward Inputs/7(Generator2_Current)  "<scaled_gcb_current>"
  Bus Selector4/3 -> Woodward Inputs/8(Mains2_Voltage)  "<scaled_mcb_voltage>"
  Bus Selector4/4 -> Woodward Inputs/9(Mains2_Current)  "<scaled_mcb_current>"
  Bus Selector4/5 -> Woodward Inputs/10(MPU2_speed)  "<scaled_speed>"
  GR1 B AIN (CH00-15)/1(Out1) -> Demux1/1
  Demux1/1 -> Bus Creator/1  "gen1_GOV_bias"
  Demux1/2 -> Bus Creator/2  "gen1_AVR_bias"
  Demux1/3 -> Bus Creator/3  "gen2_GOV_bias"
  Demux1/4 -> Bus Creator/4  "gen2_AVR_bias"
  Bus Selector5/1 -> Woodward Outputs - Diesel - Gen2/1(Gen2 MCB Status)  "<MCB_CB_Status>"
  [WoodwardBias] -> Woodward Outputs - Diesel - Gen2/2(WoodwardBias)
  [Diesel_ScaledSignals] -> Bus Selector5/1
  Woodward Outputs - Diesel - Gen2/2(Gen2 Gov and AVR) -> Bus Creator1/2  "Gov_and_AVR"
  Woodward Outputs - Diesel - Gen2/3(Gen2 Fuel Enable) -> Bus Creator1/3  "FuelEnable"
  Woodward Outputs - Diesel - Gen2/4(Gen2 GCB) -> Bus Creator1/4  "GCB_Crtl"
  Woodward Outputs - Diesel - Gen2/5(Gen2 MCB) -> Bus Creator1/5  "MCB_Ctrl"
  Bus Creator1/1 -> Bus Creator3/2  "Diesel_Gen2"
  Bus Creator3/1 -> Memory1/1
  Bus Creator2/1 -> Bus Creator3/1  "NGCHP_Gen1"
  Woodward Outputs - NGCHP - Gen1/1(Digital Inputs) -> Bus Creator2/1  "DIN"
  Woodward Outputs - NGCHP - Gen1/2(Gen1 Gov and AVR) -> Bus Creator2/2  "Gov_and_AVR"
  Woodward Outputs - NGCHP - Gen1/3(Gen1 Fuel Enable) -> Bus Creator2/3  "FuelEnable"
  Woodward Outputs - NGCHP - Gen1/4(Gen1 GCB) -> Bus Creator2/4  "GCB_Crtl"
  Woodward Outputs - Diesel - Gen2/1(Digital Inputs) -> Bus Creator1/1  "DIN"
  Woodward Outputs - NGCHP - Gen1/5(Gen1 MCB) -> Bus Creator2/5  "MCB_Ctrl"
  [WoodwardBias] -> Woodward Outputs - NGCHP - Gen1/2(WoodwardBias)
  [NGCHP_ScaledSignals] -> Bus Selector1/1
  Bus Selector1/1 -> Woodward Outputs - NGCHP - Gen1/1(Gen1 MCB Status)  "<MCB_CB_Status>"
  Memory1/1 -> WoodwardBias/1
  Bus Creator/1 -> [WoodwardBias]

== system Diesel_NGCHP_v2/SC_ctrl/RMS_Calculator5 ==
  s_in : Inport
  Demux : Demux  Outputs=3
  Discrete  Mean value6 : powerlib_extras/Discrete Measurements/Discrete  Mean value  Freq=60  Vinit=0  Ts=Ts
  Mux2 : Mux  Inputs=2
  Product3 : Product  RndMeth=Zero
  Signed Sqrt : Sqrt  SaturateOnIntegerOverflow=on
  s_out : Outport
  wires:
  Demux/1 -> Product3/1, Product3/2
  Product3/1 -> Discrete  Mean value6/1
  Discrete  Mean value6/1 -> Signed Sqrt/1
  s_in/1 -> Mux2/1, Demux/1  "3ph_inst"
  Mux2/1 -> s_out/1  "inst_rms"
  Signed Sqrt/1 -> Mux2/2  "1ph_rms"

== system Diesel_NGCHP_v2/SC_ctrl/RMS_Calculator6 ==
  s_in : Inport
  Demux : Demux  Outputs=3
  Discrete  Mean value6 : powerlib_extras/Discrete Measurements/Discrete  Mean value  Freq=60  Vinit=0  Ts=Ts
  Mux2 : Mux  Inputs=2
  Product3 : Product  RndMeth=Zero
  Signed Sqrt : Sqrt  SaturateOnIntegerOverflow=on
  s_out : Outport
  wires:
  Demux/1 -> Product3/1, Product3/2
  Product3/1 -> Discrete  Mean value6/1
  Discrete  Mean value6/1 -> Signed Sqrt/1
  s_in/1 -> Mux2/1, Demux/1  "3ph_inst"
  Mux2/1 -> s_out/1  "inst_rms"
  Signed Sqrt/1 -> Mux2/2  "1ph_rms"

== system Diesel_NGCHP_v2/SC_ctrl/RMS_Calculator7 ==
  s_in : Inport
  Demux : Demux  Outputs=3
  Discrete  Mean value6 : powerlib_extras/Discrete Measurements/Discrete  Mean value  Freq=60  Vinit=0  Ts=Ts
  Mux2 : Mux  Inputs=2
  Product3 : Product  RndMeth=Zero
  Signed Sqrt : Sqrt  SaturateOnIntegerOverflow=on
  s_out : Outport
  wires:
  Demux/1 -> Product3/1, Product3/2
  Product3/1 -> Discrete  Mean value6/1
  Discrete  Mean value6/1 -> Signed Sqrt/1
  s_in/1 -> Mux2/1, Demux/1  "3ph_inst"
  Mux2/1 -> s_out/1  "inst_rms"
  Signed Sqrt/1 -> Mux2/2  "1ph_rms"

== system Diesel_NGCHP_v2/SC_ctrl/Woodward ==
  NG_genset_data : Inport
  Diesel : Inport  Port=2
  16Din/16Dout GR3 : Subsystem
  Bus Creator1 : BusCreator  Inputs=3
  Bus Creator2 : BusCreator  Inputs=1
  Bus Creator4 : BusCreator  Inputs=3
  Bus Selector1 : BusSelector  OutputSignals=Pm,Vf,Vt,w
  Bus Selector2 : BusSelector  OutputSignals=Pm,Vf,Vt,w
  Bus Selector3 : BusSelector  OutputSignals="wref,w.wood_Gov_bias,w.Rotor speed  wm (pu)"
  Bus Selector4 : BusSelector  OutputSignals="wref,w.wood_Gov_bias,w.Rotor speed  wm (pu)"
  DieselGen : Scope  NumInputPorts=4
      settings: TimeRange=10  YMin=-0.025~-0.5~0~0  YMax=0.45~5.5~1.1~0.425
  NG-CHP : Scope  NumInputPorts=4
      settings: TimeRange=10  YMin=-0.025~-0.5~0~0  YMax=0.45~5.5~1.1~0.425  SaveName=ScopeData4
  Wood_Goiv_bias : Gain  Gain=10
  Wood_Goiv_bias1 : Gain  Gain=10
  IOctrl : Outport
  wires:
  Wood_Goiv_bias/1 -> Bus Creator4/2
  Bus Creator4/1 -> NG-CHP/4  "Speed"
  Bus Selector3/3 -> Bus Creator4/3  "<Rotor speed  wm (pu)>"
  Bus Selector3/2 -> Wood_Goiv_bias/1  "<wood_Gov_bias>"
  Bus Selector3/1 -> Bus Creator4/1  "<wref>"
  Bus Selector1/4 -> Bus Selector3/1  "<w>"
  NG_genset_data/1 -> Bus Selector1/1
  Bus Selector1/3 -> NG-CHP/3  "<Vt>"
  Bus Selector1/2 -> NG-CHP/2  "<Vf>"
  Bus Selector1/1 -> NG-CHP/1  "<Pm>"
  Wood_Goiv_bias1/1 -> Bus Creator1/2
  Bus Creator1/1 -> DieselGen/4  "Speed"
  Bus Selector4/3 -> Bus Creator1/3  "<Rotor speed  wm (pu)>"
  Bus Selector4/2 -> Wood_Goiv_bias1/1  "<wood_Gov_bias>"
  Bus Selector4/1 -> Bus Creator1/1  "<wref>"
  Bus Selector2/4 -> Bus Selector4/1  "<w>"
  Diesel/1 -> Bus Selector2/1
  Bus Selector2/3 -> DieselGen/3  "<Vt>"
  Bus Selector2/2 -> DieselGen/2  "<Vf>"
  Bus Selector2/1 -> DieselGen/1  "<Pm>"
  Bus Creator2/1 -> IOctrl/1  "IO ctrl"
  16Din/16Dout GR3/1(Dout) -> Bus Creator2/1  "16 DOUT GR3"

== system Diesel_NGCHP_v2/SM_system/4_MVA_Diesel_Generator ==
  note: This u(1)==1 is used to fix the logic problem within the woodward outputs block
  note: Copyright (c) 2016 Massachusetts Institute of Technology
      | Permission is hereby granted, free of charge, to any person obtaining a copy of this software and associated documentation files (the "Software"), to deal
      | in the Software without restriction, including without limitation the rights to use, copy, modify, merge, publish, distribute, sublicense, and/or sell copies of the
      | Software, and to permit persons to whom the Software is furnished to do so, subject to the following conditions:
      |
      | THE SOFTWARE IS PROVIDED "AS IS", WITHOUT WARRANTY OF ANY KIND, EXPRESS OR IMPLIED, INCLUDING BUT NOT LIMITED TO THE
      | WARRANTIES OF MERCHANTABILITY, FITNESS FOR A PARTICULAR PURPOSE AND NONINFRINGEMENT. IN NO EVENT SHALL THE AUTHORS
      | OR COPYRIGHT HOLDERS BE LIABLE FOR ANY CLAIM, DAMAGES OR OTHER LIABILITY, WHETHER IN AN ACTION OF CONTRACT, TORT OR
      | OTHERWISE, ARISING FROM, OUT OF OR IN CONNECTION WITH THE SOFTWARE OR THE USE OR OTHER DEALINGS IN THE SOFTWARE
  WoodwardOutputs : Inport
  Bus Creator : BusCreator  Inputs=1
  Bus Selector5 : BusSelector  OutputSignals=Diesel_Gen2.Gov_and_AVR,Diesel_Gen2.FuelEnable,Diesel_Gen2.GCB_Crtl
  Bus Selector8 : BusSelector  OutputSignals=Gen2 Ref GOV,Gen2 Ref AVR,Gen2 GOV,Gen2 AVR
  Diesel GenSet_4MVA : Subsystem  mask(Gen-Set with simulated control modes){control_mode=1}
      mask prompts: control_mode "Control Mode [0 => Sim. 1 => Wood.]"
      mask help:
      | This Gen-Set block allows the user to indicate the control mode of the generator. The available control modes are: (1) PQ, (2) PV, and (3) VF.
      | The input values to the block will be applied according to the selected control mode.
      | For example, if PQ mode is selected, the controller will only work based on P_ref and Q_ref ignoring values of other inputs to the block.
  Fcn : Fcn  Expr=u(1)==1
  ManualGenCtrl : Subsystem
  enable_woodward_control_mode_only : Constant
  Gen2 A : PMIOPort  Port=1  Side=Right
  Gen2 B : PMIOPort  Port=2  Side=Right
  Gen2 C : PMIOPort  Port=3  Side=Right
  Gen2 Monitor : Outport
  Gen2 GCB Control : Outport  Port=2
  wires:
  enable_woodward_control_mode_only/1 -> Diesel GenSet_4MVA/6(Woodward Enable)
  ManualGenCtrl/1(S) -> Diesel GenSet_4MVA/7(Manual_control)
  Diesel GenSet_4MVA/1(gen_meas) -> Gen2 Monitor/1
  Bus Selector5/1 -> Bus Selector8/1  "<Gov_and_AVR>"
  Bus Selector8/1 -> Diesel GenSet_4MVA/1(Woodward Modbus Ref for Governor)  "<Gen2 Ref GOV>"
  Bus Selector8/2 -> Diesel GenSet_4MVA/2(Woodward Modbus Ref for AVR)  "<Gen2 Ref AVR>"
  Bus Selector8/3 -> Diesel GenSet_4MVA/3(Woodward meas w)  "<Gen2 GOV>"
  Bus Selector8/4 -> Diesel GenSet_4MVA/4(Woodward meas V)  "<Gen2 AVR>"
  Bus Selector5/2 -> Diesel GenSet_4MVA/5(Generator Enable)  "<FuelEnable>"
  Fcn/1 -> Bus Creator/1  "Logic_trip"
  Bus Creator/1 -> Gen2 GCB Control/1
  Bus Selector5/3 -> Fcn/1  "<GCB_Crtl>"
  WoodwardOutputs/1 -> Bus Selector5/1
  connections:
  Gen2 A/RConn1 -- Diesel GenSet_4MVA/RConn1
  Diesel GenSet_4MVA/RConn2 -- Gen2 B/RConn1
  Gen2 C/RConn1 -- Diesel GenSet_4MVA/RConn3

== system Diesel_NGCHP_v2/SM_system/Genset_signal_scaling - 3.5MVA ==
  note: GCB V(bus) and I
  note: MCB V(line) and I
  note: Scaling for voltages:
      | For 120 => 12Vout / 170Vpk
      | For 480 => 12Vout / 391Vpk
      | For 13.8kv => 12Vout / 11268Vpk
      |
      | Scaling for currents - used in the 1 MVA genset:
      | 15Vout / ( 900,000W / 391Vpk)
      |
      | Scaling for currents - used in the 3.5 MVA NG/CHP:
      | 15Vout/( 3,150,000W / 11268Vpk)
      | --- Current scale factors chosen to match easYgen settings for 3.5 MVA gas engine CT ratio of 1500/x made on 20160508
  note: Copyright (c) 2016 Massachusetts Institute of Technology
      | Permission is hereby granted, free of charge, to any person obtaining a copy of this software and associated documentation files (the "Software"), to deal
      | in the Software without restriction, including without limitation the rights to use, copy, modify, merge, publish, distribute, sublicense, and/or sell copies of the
      | Software, and to permit persons to whom the Software is furnished to do so, subject to the following conditions:
      |
      | THE SOFTWARE IS PROVIDED "AS IS", WITHOUT WARRANTY OF ANY KIND, EXPRESS OR IMPLIED, INCLUDING BUT NOT LIMITED TO THE
      | WARRANTIES OF MERCHANTABILITY, FITNESS FOR A PARTICULAR PURPOSE AND NONINFRINGEMENT. IN NO EVENT SHALL THE AUTHORS
      | OR COPYRIGHT HOLDERS BE LIABLE FOR ANY CLAIM, DAMAGES OR OTHER LIABILITY, WHETHER IN AN ACTION OF CONTRACT, TORT OR
      | OTHERWISE, ARISING FROM, OUT OF OR IN CONNECTION WITH THE SOFTWARE OR THE USE OR OTHER DEALINGS IN THE SOFTWARE
  GCB_MS : Inport
  MCB_MS : Inport  Port=2
  MachineSpeedWm [pu] : Inport  Port=3
  Add : Sum  Inputs=+-
  Bus Creator4 : BusCreator  Inputs=6
  Bus Selector : BusSelector  OutputSignals=Status
  Bus Selector1 : BusSelector  OutputSignals=Vabc_bus,Iabc
  Bus Selector4 : BusSelector  OutputSignals=Vabc_line,Iabc
  Gain : Gain  Gain=15/Vpk_gcb
  Gain1 : Gain  Gain=15/(watt_gcb/Vpk_gcb)
  Gain2 : Gain  Gain=15/Vpk_mcb
  Gain3 : Gain  Gain=15/(watt_mcb/Vpk_mcb)
  Gain4 : Gain
  Speed_System : Subsystem  mask{rated_rpm=rated_rpm}
      mask prompts: rated_rpm "Machine Rated Speed [RPM]"
  This value is added due to the noise in the signal or the model speed6 : Constant  Value=wm_noise_bias
  ScaledSignals : Outport
  wires:
  This value is added due to the noise in the signal or the model speed6/1 -> Add/2
  MachineSpeedWm [pu]/1 -> Add/1
  GCB_MS/1 -> Bus Selector1/1
  MCB_MS/1 -> Bus Selector4/1, Bus Selector/1
  Add/1 -> Speed_System/1(wm)
  Bus Selector1/1 -> Gain/1  "<Vabc_bus>"
  Bus Selector1/2 -> Gain1/1  "<Iabc>"
  Gain3/1 -> Bus Creator4/4  "scaled_mcb_current"
  Bus Selector4/2 -> Gain3/1  "<Iabc>"
  Bus Selector4/1 -> Gain2/1  "<Vabc_line>"
  Bus Creator4/1 -> ScaledSignals/1
  Gain2/1 -> Bus Creator4/3  "scaled_mcb_voltage"
  Speed_System/1(rpm) -> Bus Creator4/5  "scaled_speed"
  Gain1/1 -> Bus Creator4/2  "scaled_gcb_current"
  Gain/1 -> Bus Creator4/1  "scaled_gcb_voltage"
  Gain4/1 -> Bus Creator4/6  "MCB_CB_Status"
  Bus Selector/1 -> Gain4/1  "<Status>"

== system Diesel_NGCHP_v2/SM_system/Genset_signal_scaling - 3.5MVA1 ==
  note: Copyright (c) 2016 Massachusetts Institute of Technology
      | Permission is hereby granted, free of charge, to any person obtaining a copy of this software and associated documentation files (the "Software"), to deal
      | in the Software without restriction, including without limitation the rights to use, copy, modify, merge, publish, distribute, sublicense, and/or sell copies of the
      | Software, and to permit persons to whom the Software is furnished to do so, subject to the following conditions:
      |
      | THE SOFTWARE IS PROVIDED "AS IS", WITHOUT WARRANTY OF ANY KIND, EXPRESS OR IMPLIED, INCLUDING BUT NOT LIMITED TO THE
      | WARRANTIES OF MERCHANTABILITY, FITNESS FOR A PARTICULAR PURPOSE AND NONINFRINGEMENT. IN NO EVENT SHALL THE AUTHORS
      | OR COPYRIGHT HOLDERS BE LIABLE FOR ANY CLAIM, DAMAGES OR OTHER LIABILITY, WHETHER IN AN ACTION OF CONTRACT, TORT OR
      | OTHERWISE, ARISING FROM, OUT OF OR IN CONNECTION WITH THE SOFTWARE OR THE USE OR OTHER DEALINGS IN THE SOFTWARE
  note: Scaling for voltages:
      | For 120 => 12Vout / 170Vpk
      | For 480 => 12Vout / 391Vpk
      | For 13.8kv => 12Vout / 11268Vpk
      |
      | Scaling for currents - used in the 1 MVA genset:
      | 15Vout / ( 900,000W / 391Vpk)
      |
      | Scaling for currents - used in the 3.5 MVA NG/CHP:
      | 15Vout/( 3,150,000W / 11268Vpk)
      | --- Current scale factors chosen to match easYgen settings for 3.5 MVA gas engine CT ratio of 1500/x made on 20160508
  note: MCB V(line) and I
  note: GCB V(bus) and I
  GCB_MS : Inport
  MCB_MS : Inport  Port=2
  MachineSpeedWm [pu] : Inport  Port=3
  Add : Sum  Inputs=+-
  Bus Creator4 : BusCreator  Inputs=6
  Bus Selector : BusSelector  OutputSignals=Status
  Bus Selector1 : BusSelector  OutputSignals=Vabc_bus,Iabc
  Bus Selector4 : BusSelector  OutputSignals=Vabc_line,Iabc
  Gain : Gain  Gain=15/Vpk_gcb
  Gain1 : Gain  Gain=15/(watt_gcb/Vpk_gcb)
  Gain2 : Gain  Gain=15/Vpk_mcb
  Gain3 : Gain  Gain=15/(watt_mcb/Vpk_mcb)
  Gain4 : Gain
  Speed_System : Subsystem  mask{rated_rpm=rated_rpm}
      mask prompts: rated_rpm "Machine Rated Speed [RPM]"
  This value is added due to the noise in the signal or the model speed6 : Constant  Value=wm_noise_bias
  ScaledSignals : Outport
  wires:
  Bus Selector/1 -> Gain4/1  "<Status>"
  Gain4/1 -> Bus Creator4/6  "MCB_CB_Status"
  Gain/1 -> Bus Creator4/1  "scaled_gcb_voltage"
  Gain1/1 -> Bus Creator4/2  "scaled_gcb_current"
  Speed_System/1(rpm) -> Bus Creator4/5  "scaled_speed"
  Gain2/1 -> Bus Creator4/3  "scaled_mcb_voltage"
  Bus Creator4/1 -> ScaledSignals/1
  Bus Selector4/1 -> Gain2/1  "<Vabc_line>"
  Bus Selector4/2 -> Gain3/1  "<Iabc>"
  Gain3/1 -> Bus Creator4/4  "scaled_mcb_current"
  Bus Selector1/2 -> Gain1/1  "<Iabc>"
  Bus Selector1/1 -> Gain/1  "<Vabc_bus>"
  Add/1 -> Speed_System/1(wm)
  MCB_MS/1 -> Bus Selector/1, Bus Selector4/1
  GCB_MS/1 -> Bus Selector1/1
  MachineSpeedWm [pu]/1 -> Add/1
  This value is added due to the noise in the signal or the model speed6/1 -> Add/2

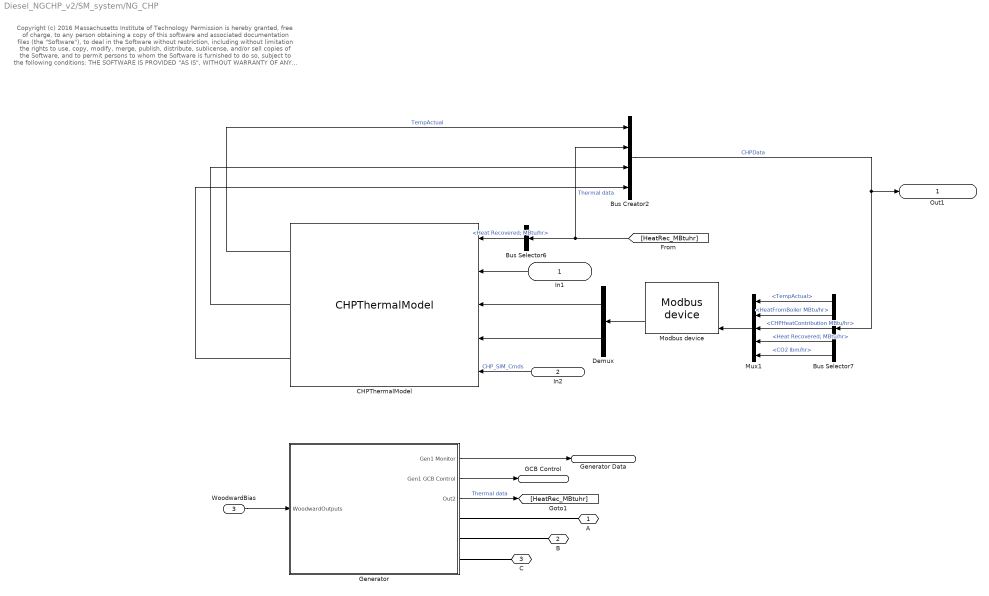
== system Diesel_NGCHP_v2/SM_system/NG_CHP ==
  note: Copyright (c) 2016 Massachusetts Institute of Technology
      | Permission is hereby granted, free of charge, to any person obtaining a copy of this software and associated documentation files (the "Software"), to deal
      | in the Software without restriction, including without limitation the rights to use, copy, modify, merge, publish, distribute, sublicense, and/or sell copies of the
      | Software, and to permit persons to whom the Software is furnished to do so, subject to the following conditions:
      |
      | THE SOFTWARE IS PROVIDED "AS IS", WITHOUT WARRANTY OF ANY KIND, EXPRESS OR IMPLIED, INCLUDING BUT NOT LIMITED TO THE
      | WARRANTIES OF MERCHANTABILITY, FITNESS FOR A PARTICULAR PURPOSE AND NONINFRINGEMENT. IN NO EVENT SHALL THE AUTHORS
      | OR COPYRIGHT HOLDERS BE LIABLE FOR ANY CLAIM, DAMAGES OR OTHER LIABILITY, WHETHER IN AN ACTION OF CONTRACT, TORT OR
      | OTHERWISE, ARISING FROM, OUT OF OR IN CONNECTION WITH THE SOFTWARE OR THE USE OR OTHER DEALINGS IN THE SOFTWARE
  In1 : Inport
  In2 : Inport  Port=2
  WoodwardBias : Inport  Port=3
  Bus Creator2 : BusCreator
  Bus Selector6 : BusSelector  OutputSignals=Heat Recovered; MBtu/hr
  Bus Selector7 : BusSelector  OutputSignals=TempActual,HeatFromBoiler MBtu/hr,CHPHeatContribution MBtu/hr,Thermal data.Heat Recovered; MBtu/hr,Thermal data.CO2 lbm/hr
  CHPThermalModel : CHP_Model_lib/CHPThermalModel  SIM_HIL=SIM_HIL
  Demux : Demux  Outputs=2
  Generator : Subsystem  AncestorBlock=NG_Genset_lib/Generator
  Modbus device : rtio_generic_modbus/Modbus device  conf_name=CHP_slave_cfg.opal  conf_name_mask=CHP_slave_cfg.xls  sample_time=Ts
  Mux1 : Mux  Inputs=5
  A : PMIOPort  Tag=A  Port=1  Side=Right
      settings: AttributesFormatString=A
  B : PMIOPort  Port=2  Side=Right
  C : PMIOPort  Port=3  Side=Right
  Out1 : Outport
  Generator Data : Outport  Port=2
  GCB Control : Outport  Port=3
  wires:
  In2/1 -> CHPThermalModel/5  "CHP_SIM_Cmds"
  Bus Creator2/1 -> Out1/1, Bus Selector7/1  "CHPData"
  Bus Selector6/1 -> CHPThermalModel/1  "<Heat Recovered; MBtu/hr>"
  Generator/2(Gen1 GCB Control) -> GCB Control/1
  Generator/1(Gen1 Monitor) -> Generator Data/1
  Modbus device/2 -> Demux/1
  [HeatRec_MBtuhr] -> Bus Selector6/1, Bus Creator2/2  "Thermal data"
  CHPThermalModel/3 -> Bus Creator2/4
  Demux/1 -> CHPThermalModel/3
  Mux1/1 -> Modbus device/4
  In1/1 -> CHPThermalModel/2
  Bus Selector7/1 -> Mux1/1  "<TempActual>"
  Bus Selector7/4 -> Mux1/4  "<Heat Recovered; MBtu/hr>"
  Bus Selector7/5 -> Mux1/5  "<CO2 lbm/hr>"
  Bus Selector7/2 -> Mux1/2  "<HeatFromBoiler MBtu/hr>"
  CHPThermalModel/2 -> Bus Creator2/3
  Demux/2 -> CHPThermalModel/4
  CHPThermalModel/1 -> Bus Creator2/1  "TempActual"
  Bus Selector7/3 -> Mux1/3  "<CHPHeatContribution MBtu/hr>"
  Generator/3(Out2) -> [HeatRec_MBtuhr]  "Thermal data"
  WoodwardBias/1 -> Generator/1(WoodwardOutputs)
  connections:
  Generator/RConn1 -- A/RConn1
  Generator/RConn2 -- B/RConn1
  Generator/RConn3 -- C/RConn1

== system Diesel_NGCHP_v2/SS_signals/GR1 B AIN (CH00-15) ==
  AnalogIn : rtio_opalrt_common/AnalogIn  CtrlName='OpCtrl'  portNb=1  FcnNos=Slot 0 Module X Subsection 0  size=16  maxcount=0  count=8  numchan=8  sampleTime=0
      settings: AttributesFormatString=%<CtrlName>
  AnalogIn1 : rtio_opalrt_common/AnalogIn  CtrlName='OpCtrl'  portNb=2  FcnNos=Slot 0 Module X Subsection 0  size=16  maxcount=0  count=8  numchan=8  sampleTime=0
      settings: AttributesFormatString=%<CtrlName>
  Mux6 : Mux  Inputs=2
  Terminator2 : Terminator
  Terminator3 : Terminator
  Out1 : Outport
  wires:
  AnalogIn/1 -> Mux6/1
  AnalogIn1/1 -> Mux6/2
  AnalogIn/2 -> Terminator2/1
  AnalogIn1/2 -> Terminator3/1
  Mux6/1 -> Out1/1

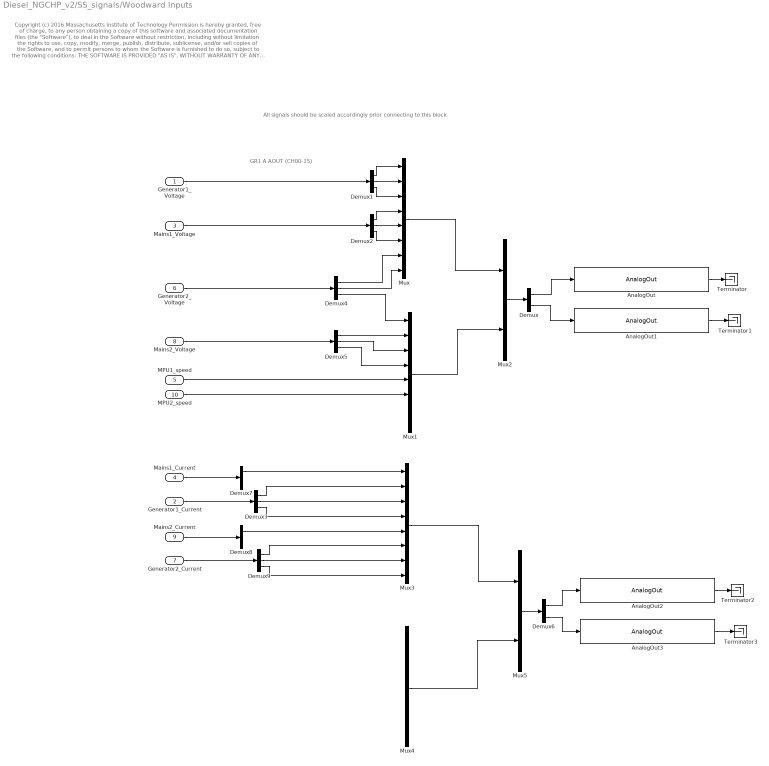
== system Diesel_NGCHP_v2/SS_signals/Woodward Inputs ==
  note: All signals should be scaled accordingly prior connecting to this block
  note: GR1 A AOUT (CH00-15)
  note: Copyright (c) 2016 Massachusetts Institute of Technology
      | Permission is hereby granted, free of charge, to any person obtaining a copy of this software and associated documentation files (the "Software"), to deal
      | in the Software without restriction, including without limitation the rights to use, copy, modify, merge, publish, distribute, sublicense, and/or sell copies of the
      | Software, and to permit persons to whom the Software is furnished to do so, subject to the following conditions:
      |
      | THE SOFTWARE IS PROVIDED "AS IS", WITHOUT WARRANTY OF ANY KIND, EXPRESS OR IMPLIED, INCLUDING BUT NOT LIMITED TO THE
      | WARRANTIES OF MERCHANTABILITY, FITNESS FOR A PARTICULAR PURPOSE AND NONINFRINGEMENT. IN NO EVENT SHALL THE AUTHORS
      | OR COPYRIGHT HOLDERS BE LIABLE FOR ANY CLAIM, DAMAGES OR OTHER LIABILITY, WHETHER IN AN ACTION OF CONTRACT, TORT OR
      | OTHERWISE, ARISING FROM, OUT OF OR IN CONNECTION WITH THE SOFTWARE OR THE USE OR OTHER DEALINGS IN THE SOFTWARE
  Generator1_Voltage : Inport
  Generator1_Current : Inport  Port=2
  Mains1_Voltage : Inport  Port=3
  Mains1_Current : Inport  Port=4
  MPU1_speed : Inport  Port=5
  Generator2_Voltage : Inport  Port=6
  Generator2_Current : Inport  Port=7
  Mains2_Voltage : Inport  Port=8
  Mains2_Current : Inport  Port=9
  MPU2_speed : Inport  Port=10
  AnalogOut : rtio_opalrt_common/AnalogOut  CtrlName='OpCtrl'  portNb=1  FcnNos=Slot 0 Module X Subsection 0  size=16  maxcount=-2  count=-2  numchan=8  israngeinput=off  voltagerange=[-16 ... 16]  slot=0  side=0  mismatch=0  slotside=Slot_1_Module_A
      settings: AttributesFormatString=%<CtrlName>
  AnalogOut1 : rtio_opalrt_common/AnalogOut  CtrlName='OpCtrl'  portNb=2  FcnNos=Slot 0 Module X Subsection 0  size=16  maxcount=-2  count=-2  numchan=8  israngeinput=off  voltagerange=[-16 ... 16]  slot=0  side=0  mismatch=0  slotside=Slot_1_Module_A
      settings: AttributesFormatString=%<CtrlName>
  AnalogOut2 : rtio_opalrt_common/AnalogOut  CtrlName='OpCtrl'  portNb=3  FcnNos=Slot 0 Module X Subsection 0  size=16  maxcount=-2  count=-2  numchan=8  israngeinput=off  voltagerange=[-16 ... 16]  slot=1  side=0  mismatch=0  slotside=Slot_2_Module_A
      settings: AttributesFormatString=%<CtrlName>
  AnalogOut3 : rtio_opalrt_common/AnalogOut  CtrlName='OpCtrl'  portNb=4  FcnNos=Slot 0 Module X Subsection 0  size=16  maxcount=-2  count=-2  numchan=8  israngeinput=off  voltagerange=[-16 ... 16]  slot=1  side=0  mismatch=0  slotside=Slot_2_Module_A
      settings: AttributesFormatString=%<CtrlName>
  Demux : Demux  Outputs=2
  Demux{1..5,7..9} (8 alike) : Demux  Outputs=3
  Demux6 : Demux  Outputs=2
  Mux{,1,3..4} (4 alike) : Mux  Inputs=8
  Mux2 : Mux  Inputs=2
  Mux5 : Mux  Inputs=2
  Terminator{,1..3} (4 alike) : Terminator
  wires:
  Demux9/3 -> Mux3/8
  Demux9/2 -> Mux3/7
  Demux9/1 -> Mux3/6
  Generator2_Current/1 -> Demux9/1
  Demux8/1 -> Mux3/5
  Mains2_Current/1 -> Demux8/1
  MPU2_speed/1 -> Mux1/6
  Generator2_Voltage/1 -> Demux4/1
  Mains2_Voltage/1 -> Demux5/1
  Demux7/1 -> Mux3/1
  Mains1_Current/1 -> Demux7/1
  Demux3/3 -> Mux3/4
  Demux3/2 -> Mux3/3
  Demux3/1 -> Mux3/2
  Generator1_Current/1 -> Demux3/1
  AnalogOut2/1 -> Terminator2/1
  AnalogOut3/1 -> Terminator3/1
  Demux6/1 -> AnalogOut2/1
  Demux6/2 -> AnalogOut3/1
  Mux3/1 -> Mux5/1
  Mux4/1 -> Mux5/2
  Mux5/1 -> Demux6/1
  Demux5/3 -> Mux1/4
  Demux5/2 -> Mux1/3
  Demux5/1 -> Mux1/2
  Demux4/3 -> Mux1/1
  Demux4/2 -> Mux/8
  Demux4/1 -> Mux/7
  MPU1_speed/1 -> Mux1/5
  Demux2/3 -> Mux/6
  Demux2/2 -> Mux/5
  Demux2/1 -> Mux/4
  Demux1/3 -> Mux/3
  Demux1/2 -> Mux/2
  Demux1/1 -> Mux/1
  AnalogOut/1 -> Terminator/1
  AnalogOut1/1 -> Terminator1/1
  Demux/1 -> AnalogOut/1
  Demux/2 -> AnalogOut1/1
  Mux/1 -> Mux2/1
  Mux1/1 -> Mux2/2
  Mux2/1 -> Demux/1
  Generator1_Voltage/1 -> Demux1/1
  Mains1_Voltage/1 -> Demux2/1
